simulink model "Filter_Reference"  (R2020b)
settings: Solver=FixedStepAuto  StartTime=0.0  StopTime=10.0  FixedStep=0.2  RelTol=1e-3
settings Model: Creator=Shirish  LastModifiedBy=Shirish
settings DataIOCC: SaveOutput=off  SaveTime=off

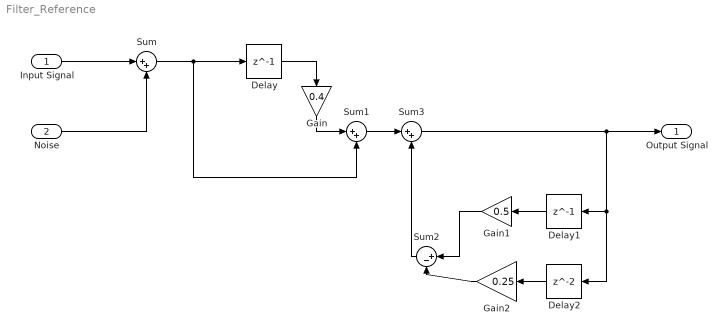
== system Filter_Reference ==
  Input Signal : Inport  OutDataTypeStr=double  PortDimensions=1  SampleTime=[0.20000000000000001,0]
  Noise : Inport  Port=2  OutDataTypeStr=double  PortDimensions=1  SampleTime=[0.20000000000000001,0]
  Delay : Delay  DelayLength=1
  Delay1 : Delay  DelayLength=1
  Delay2 : Delay
  Gain : Gain  Gain=0.4
  Gain1 : Gain  Gain=0.5
  Gain2 : Gain  Gain=0.25
  Sum : Sum  Inputs=|++
  Sum1 : Sum  Inputs=|++
  Sum2 : Sum  Inputs=|+-
  Sum3 : Sum  Inputs=|++
  Output Signal : Outport  OutDataTypeStr=double  PortDimensions=1  SampleTime=[0.20000000000000001,0]
  wires:
  Gain1/1 -> Sum2/1
  Sum/1 -> Delay/1, Sum1/2
  Delay1/1 -> Gain1/1
  Gain/1 -> Sum1/1
  Delay/1 -> Gain/1
  Sum2/1 -> Sum3/2
  Sum1/1 -> Sum3/1
  Sum3/1 -> Delay1/1, Delay2/1, Output Signal/1
  Delay2/1 -> Gain2/1
  Noise/1 -> Sum/2
  Gain2/1 -> Sum2/2
  Input Signal/1 -> Sum/1
